simulink model "design_sl"  (R2023b)
settings: Solver=VariableStepAuto  StartTime=0.0  StopTime=3  RelTol=1e-3
undefined symbols (not defined in the file or in its folder): arrayFinalDen, arrayFinalNum
libraries: spsTriangleGeneratorLib x1
settings Model: Creator=camil  LastModifiedBy=camil

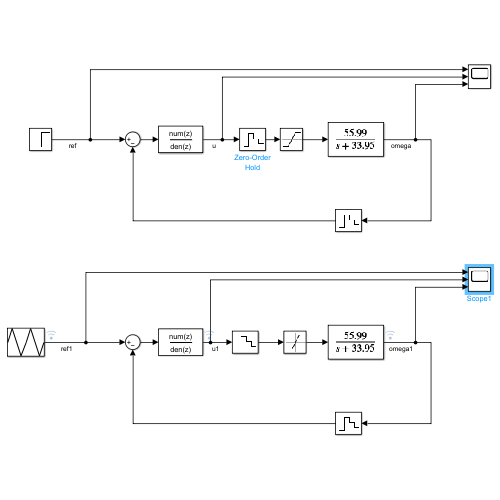
[thumbnail: Simulink's stored preview of the top-level diagram]
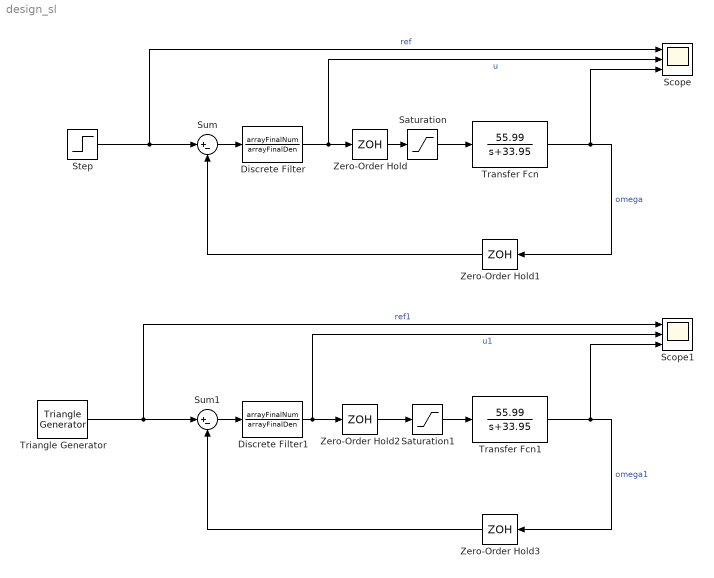
== system design_sl ==
  Discrete Filter : DiscreteFilter  Numerator=arrayFinalNum  Denominator=arrayFinalDen
  Discrete Filter1 : DiscreteFilter  Numerator=arrayFinalNum  Denominator=arrayFinalDen
  Saturation : Saturate  UpperLimit=1  LowerLimit=-1
  Saturation1 : Saturate  UpperLimit=1  LowerLimit=-1
  Scope : Scope  NumInputPorts=3
  Scope1 : Scope  NumInputPorts=3
  Step : Step  SampleTime=0.005
  Sum : Sum  Inputs=|+-
  Sum1 : Sum  Inputs=|+-
  Transfer Fcn : TransferFcn  Numerator=[55.99]  Denominator=[1 33.95]
  Transfer Fcn1 : TransferFcn  Numerator=[55.99]  Denominator=[1 33.95]
  Triangle Generator : spsTriangleGeneratorLib/Triangle Generator  Freq=0.5  Phase=90  Ts=0.005
  Zero-Order Hold{,1..3} (4 alike) : ZeroOrderHold  SampleTime=0.005
  wires:
  Discrete Filter/1 -> Scope/2, Zero-Order Hold/1  "u"
  Transfer Fcn/1 -> Scope/3, Zero-Order Hold1/1  "omega"
  Step/1 -> Sum/1, Scope/1  "ref"
  Sum/1 -> Discrete Filter/1
  Saturation/1 -> Transfer Fcn/1
  Zero-Order Hold/1 -> Saturation/1
  Zero-Order Hold1/1 -> Sum/2
  Zero-Order Hold2/1 -> Saturation1/1
  Discrete Filter1/1 -> Scope1/2, Zero-Order Hold2/1  "u1"
  Zero-Order Hold3/1 -> Sum1/2
  Triangle Generator/1 -> Sum1/1, Scope1/1  "ref1"
  Sum1/1 -> Discrete Filter1/1
  Transfer Fcn1/1 -> Scope1/3, Zero-Order Hold3/1  "omega1"
  Saturation1/1 -> Transfer Fcn1/1
